simulink subsystem "Experimental_Control"  (R2025a)
settings: Solver=VariableStepAuto  StartTime=0.0  StopTime=10.0  RelTol=1e-3
settings Model: Creator=gurt1  LastModifiedBy=gurt1

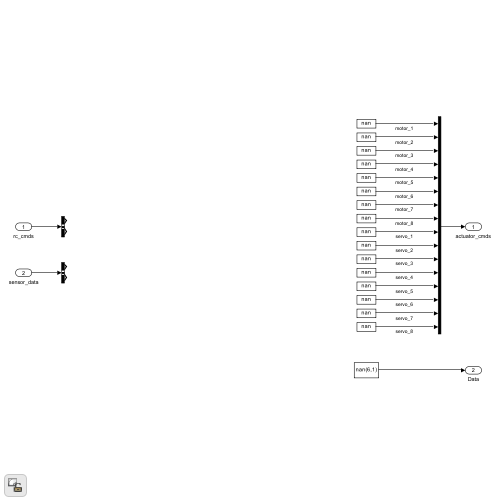
[thumbnail: Simulink's stored preview of the top-level diagram]
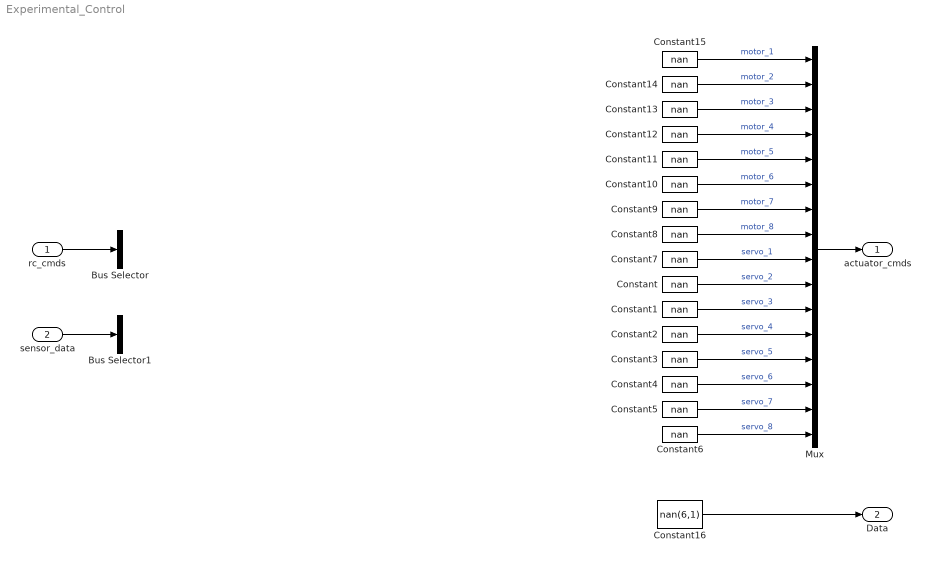
== system Experimental_Control ==
  rc_cmds : Inport
  sensor_data : Inport  Port=2
  Bus Selector : BusSelector  OutputSignals=signal1,signal2
  Bus Selector1 : BusSelector  OutputSignals=signal1,signal2
  Constant{,1..15} (16 alike) : Constant  Value=nan
  Constant16 : Constant  Value=nan(6,1)
  Mux : Mux  Inputs=16
  actuator_cmds : Outport
  Data : Outport  Port=2
  wires:
  sensor_data/1 -> Bus Selector1/1
  rc_cmds/1 -> Bus Selector/1
  Mux/1 -> actuator_cmds/1
  Constant14/1 -> Mux/2  "motor_2"
  Constant8/1 -> Mux/8  "motor_8"
  Constant5/1 -> Mux/15  "servo_7"
  Constant/1 -> Mux/10  "servo_2"
  Constant2/1 -> Mux/12  "servo_4"
  Constant10/1 -> Mux/6  "motor_6"
  Constant9/1 -> Mux/7  "motor_7"
  Constant1/1 -> Mux/11  "servo_3"
  Constant15/1 -> Mux/1  "motor_1"
  Constant4/1 -> Mux/14  "servo_6"
  Constant13/1 -> Mux/3  "motor_3"
  Constant11/1 -> Mux/5  "motor_5"
  Constant12/1 -> Mux/4  "motor_4"
  Constant7/1 -> Mux/9  "servo_1"
  Constant6/1 -> Mux/16  "servo_8"
  Constant3/1 -> Mux/13  "servo_5"
  Constant16/1 -> Data/1
